simulink model "three_phase_csi"  (Simulink 6.1)
settings: Solver=ode23tb  SolverMode=SingleTasking  StartTime=0.0  StopTime=0.2  RelTol=1e-3
libraries: powerlib x14
settings Model: Creator=patrice  LastModifiedBy=ThinkPad  ExtModeTrigMode=oneshot  ExtModeArmWhenConnect=off  ExtModeAutoUpdateStatusClock=off
settings DataIOCC: LimitDataPoints=off  SignalLoggingName=sigsOut
settings OptimizationCC: BooleanDataType=off
settings HardwareCC: TargetUnknown=on
settings RTWCC: TemplateMakefile=grt_unix.tmf

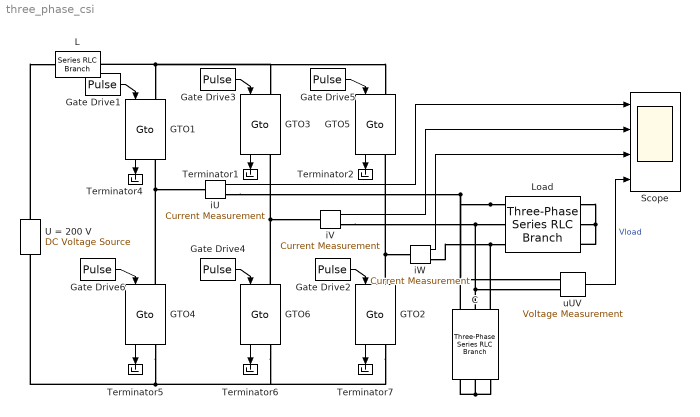
== system three_phase_csi ==
  C : powerlib/Elements/Three-Phase Series RLC Branch  Orientation=up  PhysicalDomain=powersysdomain  SubClassName=unknown  LeftPortType=p1  RightPortType=p1  LConnTagsString=A|B|C  RConnTagsString=A|B|C  Resistance=0  Inductance=0  Capacitance=1e-4  Measurements=None
  GTO{1..6} (6 alike) : powerlib/Power Electronics/Gto  Orientation=down  Ron=0.01  Lon=1e-6  Vf=1  Tf=10e-6  Tt=20e-6  IC=0  Rs=100  Cs=1e-6  Measurements=on
      settings: AttributesFormatString=\n
  Gate Drive1 : DiscretePulseGenerator  PulseType=Time based  Period=0.02  PulseWidth=33.4
  Gate Drive2 : DiscretePulseGenerator  PulseType=Time based  Period=0.02  PulseWidth=33.4  PhaseDelay=0.00333
  Gate Drive3 : DiscretePulseGenerator  PulseType=Time based  Period=0.02  PulseWidth=33.4  PhaseDelay=0.00667
  Gate Drive4 : DiscretePulseGenerator  PulseType=Time based  Period=0.02  PulseWidth=33.4  PhaseDelay=0.01667
  Gate Drive5 : DiscretePulseGenerator  PulseType=Time based  Period=0.02  PulseWidth=33.4  PhaseDelay=0.01333
  Gate Drive6 : DiscretePulseGenerator  PulseType=Time based  Period=0.02  PulseWidth=33.4  PhaseDelay=0.01
  L : powerlib/Elements/Series RLC Branch  Orientation=left  PhysicalDomain=powersysdomain  SubClassName=unknown  LeftPortType=p1  RightPortType=p1  LConnTagsString=__new0  RConnTagsString=__new0  Resistance=0  Inductance=2e-02  Capacitance=inf  Measurements=None
  Load : powerlib/Elements/Three-Phase Series RLC Branch  PhysicalDomain=powersysdomain  SubClassName=unknown  LeftPortType=p1  RightPortType=p1  LConnTagsString=A|B|C  RConnTagsString=A|B|C  Resistance=8  Inductance=5e-3  Capacitance=inf  Measurements=None
  Scope : Scope  NumInputPorts=4
      settings: TimeRange=0.1  YMin=-20~-20~-20~-400  YMax=20~20~20~400
  Terminator{1..2,4..7} (6 alike) : Terminator
      settings: Orientation=down
  U = 200 V : powerlib/Electrical Sources/DC Voltage Source  Description=source block  Orientation=up  Amplitude=200  Measurements=None
      settings: AttributesFormatString=\n
  iU : powerlib/Measurements/Current Measurement  Tag=PoWeRsYsTeMmEaSuReMeNt  PhasorSimulation=off  OutputType=Magnitude  PSBequivalent=0
  iV : powerlib/Measurements/Current Measurement  Tag=PoWeRsYsTeMmEaSuReMeNt  PhasorSimulation=off  OutputType=Magnitude  PSBequivalent=0
  iW : powerlib/Measurements/Current Measurement  Tag=PoWeRsYsTeMmEaSuReMeNt  PhasorSimulation=off  OutputType=Magnitude  PSBequivalent=0
  uUV : powerlib/Measurements/Voltage Measurement  Tag=PoWeRsYsTeMmEaSuReMeNt  PhasorSimulation=off  OutputType=Magnitude  PSBequivalent=0
  wires:
  uUV/1 -> Scope/4  "Vload"
  Gate Drive1/1 -> GTO1/1
  Gate Drive3/1 -> GTO3/1
  Gate Drive5/1 -> GTO5/1
  Gate Drive2/1 -> GTO2/1
  Gate Drive4/1 -> GTO6/1
  Gate Drive6/1 -> GTO4/1
  iU/1 -> Scope/1
  iV/1 -> Scope/2
  iW/1 -> Scope/3
  GTO4/1 -> Terminator5/1
  GTO6/1 -> Terminator6/1
  GTO2/1 -> Terminator7/1
  GTO1/1 -> Terminator4/1
  GTO3/1 -> Terminator1/1
  GTO5/1 -> Terminator2/1
  connections:
  GTO2/RConn1 -- GTO6/RConn1 -- U = 200 V/LConn1 -- GTO4/RConn1
  U = 200 V/RConn1 -- L/RConn1
  GTO5/LConn1 -- GTO3/LConn1 -- GTO1/LConn1 -- L/LConn1
  Load/LConn1 -- iU/RConn1 -- C/RConn1 -- uUV/LConn1
  C/RConn2 -- Load/LConn2 -- iV/RConn1 -- uUV/LConn2
  C/RConn3 -- Load/LConn3 -- iW/RConn1
  Load/RConn1 -- Load/RConn3 -- Load/RConn2
  GTO4/LConn1 -- GTO1/RConn1 -- iU/LConn1
  GTO2/LConn1 -- GTO5/RConn1 -- iW/LConn1
  GTO6/LConn1 -- GTO3/RConn1 -- iV/LConn1
  C/LConn3 -- C/LConn1 -- C/LConn2
